simulink model "bObserver"  (R2020a)
settings: Solver=VariableStepAuto  StartTime=0.0  StopTime=1.5  FixedStep=0.0005  EnableMultiTasking=on
InitFcn:
  | kp=0.01;
  | ki=0.01;
  | 
  | k=2;
  | em=100000000;
  | GE=1/em;
  | GU=k*ki/GE;
  | GCE=k*kp/GU;
model workspace (MAT data in the model file):
  time = 0.8
values from neighbouring files (symbols this model uses):
  A1 = obj.boostConverter.A1    [BoostController.m]    (also in BoostConverter.m = [-obj.R/obj.L 0;0 -1/(obj.Ro*obj.C)]; BuckBoostConverter.m = [-obj.R/obj.L 0;0 -1/(obj.Ro*obj.C)]; obsmc.m = Asigma{1,1}; workspace_atual.mat = [-16.4  0; 0  -3.50877192982])
  A2 = obj.boostConverter.A2    [BoostController.m]    (also in BoostConverter.m = [-obj.R/obj.L -1/obj.L;1/obj.C -1/(obj.Ro*obj.C)]; BuckBoostConverter.m = [-obj.R/obj.L 1/obj.L;-1/obj.C -1/(obj.Ro*obj.C)]; obsmc.m = Asigma{1,2}; workspace_atual.mat = [-16.4  -200; 350.877192982  -3.50877192982])
  AlarmDeadTime = 0.50    (= 0.5)    [BoostFaultSimulation.m]    (also in workspace_atual.mat; workspace_certo.mat)
  B1 = obj.boostConverter.B1    [BoostController.m]    (also in BoostConverter.m = [1/obj.L;0]; BuckBoostConverter.m = [1/obj.L;0]; obsmc.m = Bsigma{1,1}; workspace_atual.mat = [200 0])
  B1f = [200 0]    [workspace_atual.mat]    (also in workspace_certo.mat)
  B2 = obj.boostConverter.B2    [BoostController.m]    (also in BoostConverter.m = obj.B1; obsmc.m = Bsigma{1,2}; workspace_atual.mat = [200 0]; workspace_certo.mat = [200 0])
  B2f = [200 0]    [workspace_atual.mat]    (also in workspace_certo.mat)
  boost_Amatrices = cat(3,obj.A1,obj.A2)    [BoostConverter.m]    (also in BuckBoostConverter.m; boostResults2Latex.m = boost.A_matrices(); workspace_atual.mat = [-16.4 0 0 -3.50877192982 -16.4 350.877192982 -200 -3.508771; workspace_certo.mat = [-16.4 0 0 -3.50877192982 -16.4 350.877192982 -200 -3.508771)
  boost_parameters = [obj.Ro,obj.R,obj.L,obj.C,obj.u]'    [BoostConverter.m]    (also in BuckBoostConverter.m; boostResults2Latex.m = boost.parameters(); workspace_atual.mat = [100 0.082 0.005 0.00285 190]; workspace_certo.mat = [100 0.082 0.005 0.00285 190])
  C = 1e-3    (= 0.001)    [boostResults2Latex.m]
  CiL = [0 1]    [workspace_atual.mat]    (also in workspace_certo.mat)
  Cmatrix = [1  0; 0  1]    [workspace_atual.mat]    (also in workspace_certo.mat)
  CVc = [1 0]    [workspace_atual.mat]    (also in workspace_certo.mat)
  D1 = [1  0; 0  1]    [workspace_atual.mat]    (also in workspace_certo.mat)
  F_11 = -16.4    [workspace_atual.mat]    (also in workspace_certo.mat)
  F_12 = -4812476.87956    [workspace_atual.mat]    (also in workspace_certo.mat)
  F_21 = -3.50877192982    [workspace_atual.mat]    (also in workspace_certo.mat)
  F_22 = -2.00703596657    [workspace_atual.mat]    (also in workspace_certo.mat)
  FaultClass = 0    [BoostFaultSimulation.m]    (also in workspace_atual.mat = 1; workspace_certo.mat = 1)
  H_1 = 13715.5123667    [workspace_atual.mat]    (also in workspace_certo.mat)
  iLFaultSwitch = 0    [BoostFaultSimulation.m]    (also in workspace_atual.mat; workspace_certo.mat)
  iLFaultTime = 1.70    (= 1.7)    [BoostFaultSimulation.m]    (also in workspace_atual.mat; workspace_certo.mat)
  iLGainFaultFactor = 15    [BoostFaultSimulation.m]    (also in workspace_atual.mat; workspace_certo.mat)
  iLNoiseFaultSwitch = 0    [BoostFaultSimulation.m]    (also in workspace_atual.mat; workspace_certo.mat)
  iLNoiseTime = 1.70    (= 1.7)    [BoostFaultSimulation.m]    (also in workspace_atual.mat; workspace_certo.mat)
  Jth = 2000    [workspace_atual.mat]    (also in workspace_certo.mat)
  L = 1e-3    (= 0.001)    [boostResults2Latex.m]    (also in obsmc.m = sdpvar(3,1,'full'))
  L_11 = -176809.798019    [workspace_atual.mat]    (also in workspace_certo.mat)
  L_12 = -66005538231.6    [workspace_atual.mat]    (also in workspace_certo.mat)
  L_21 = 0.0967961040176    [workspace_atual.mat]    (also in workspace_certo.mat)
  L_22 = 350.985265141    [workspace_atual.mat]    (also in workspace_certo.mat)
  LoadAddSignalSwitch = 1    [BoostFaultSimulation.m]    (also in workspace_atual.mat; workspace_certo.mat)
  LoadAddSwitch = 0    [BoostFaultSimulation.m]    (also in workspace_atual.mat; workspace_certo.mat)
  LoadAddTime = 0.90    (= 0.9)    [BoostFaultSimulation.m]    (also in workspace_atual.mat; workspace_certo.mat)
  LoadRemoveSignalSwitch = 1    [BoostFaultSimulation.m]    (also in workspace_atual.mat; workspace_certo.mat)
  LoadRemoveSwitch = 0    [BoostFaultSimulation.m]    (also in workspace_atual.mat; workspace_certo.mat)
  LoadRemoveTime = 0.90    (= 0.9)    [BoostFaultSimulation.m]    (also in workspace_atual.mat; workspace_certo.mat)
  LobsiL = [1737913.15707 66180.0912281]    [workspace_atual.mat]    (also in workspace_certo.mat)
  LobsVc = [61200 1]    [workspace_atual.mat]    (also in workspace_certo.mat)
  ObsEp = 70    [workspace_atual.mat]    (also in workspace_certo.mat)
  P = value(P)    [BoostController.m]    (also in boostResults2Latex.m = boost.calculateP(); obsmc.m = blkdiag(1/deltaAtilde(1,2),-1/deltaAtilde(2,1),1); workspace_atual.mat = [0.00235275094895  5.25738510027e-05; 5.25738510027e-05  0.0; workspace_certo.mat = [0.00235275094893  5.25738512446e-05; 5.25738512446e-05  0.0)
  Q_1 = [13715.5123667  1; 1  0]    [workspace_atual.mat]    (also in workspace_certo.mat)
  Q_2 = [1  0; 0.00750867981628  1]    [workspace_atual.mat]    (also in workspace_certo.mat)
  R = 0.1    [boostResults2Latex.m]    (also in workspace_atual.mat = 0.082; workspace_certo.mat = 0.082)
  ReconfigSwitch = 0    [BoostFaultSimulation.m]    (also in workspace_atual.mat; workspace_certo.mat)
  ReconfigTime = 1.707    [BoostFaultSimulation.m]    (also in workspace_atual.mat; workspace_certo.mat)
  rho = 5    [workspace_atual.mat]    (also in workspace_certo.mat)
  RMSfrequency = 47.61    [BoostFaultSimulation.m]    (also in workspace_atual.mat; workspace_certo.mat)
  Ro = 100    [BoostFaultSimulation.m]    (also in boostResults2Latex.m = 10; workspace_atual.mat; workspace_certo.mat)
  Smep = 80    [workspace_atual.mat]    (also in workspace_certo.mat)
  SourceAddSignalSwitch = 1    [BoostFaultSimulation.m]    (also in workspace_atual.mat; workspace_certo.mat)
  SourceAddSwitch = 0    [BoostFaultSimulation.m]    (also in workspace_atual.mat; workspace_certo.mat)
  SourceAddTime = 0.90    (= 0.9)    [BoostFaultSimulation.m]    (also in workspace_atual.mat; workspace_certo.mat)
  SourceAddVoltage = obj.SourceAddFactor*obj.u    [BoostFaultSimulation.m]    (also in workspace_atual.mat = 19; workspace_certo.mat = 19)
  SourceRemoveSignalSwitch = 1    [BoostFaultSimulation.m]    (also in workspace_atual.mat; workspace_certo.mat)
  SourceRemoveSwitch = 0    [BoostFaultSimulation.m]    (also in workspace_atual.mat; workspace_certo.mat)
  SourceRemoveTime = 0.90    (= 0.9)    [BoostFaultSimulation.m]    (also in workspace_atual.mat; workspace_certo.mat)
  SourceRemoveVoltage = obj.SourceRemoveFactor*obj.u    [BoostFaultSimulation.m]    (also in workspace_atual.mat = 19; workspace_certo.mat = 19)
  T_1 = [1 -13715.5123667]    [workspace_atual.mat]    (also in workspace_certo.mat)
  T_2 = [-0.00750867981628 1]    [workspace_atual.mat]    (also in workspace_certo.mat)
  ueq = 0.5    [workspace_atual.mat]    (also in workspace_certo.mat)
  uf = 190    [workspace_atual.mat]    (also in workspace_certo.mat)
  VcFaultSwitch = 0    [BoostFaultSimulation.m]    (also in workspace_atual.mat; workspace_certo.mat)
  VcFaultTime = 1.70    (= 1.7)    [BoostFaultSimulation.m]    (also in workspace_atual.mat; workspace_certo.mat)
  VcGainFaultFactor = 15    [BoostFaultSimulation.m]    (also in workspace_atual.mat; workspace_certo.mat)
  VcNoiseFaultSwitch = 0    [BoostFaultSimulation.m]    (also in workspace_atual.mat; workspace_certo.mat)
  VcNoiseTime = 1.70    (= 1.7)    [BoostFaultSimulation.m]    (also in workspace_atual.mat; workspace_certo.mat)
  ve = 380    [BoostFaultSimulation.m]    (also in boostResults2Latex.m = 100; workspace_atual.mat; workspace_certo.mat)
  x_e = [ie;ve]    [BoostConverter.m]    (also in BuckBoostConverter.m)
  xe = obj.boostConverter.equilibriumstate(ve)    [BoostController.m]    (also in workspace_atual.mat = [7.62509288104 380]; workspace_certo.mat = [7.62509288104 380])
undefined symbols (not defined in the file or in its folder): Atilde1, Atilde2, B1u, Ctilde1, Dtilde1, Dtilde2, F, F1, G, G1, MAXnet, MINnet
libraries: neural x36, powerlib x34, dspstat3 x11, PhdLibrary x10, simulink x7, dspmtrx3 x6, powerlib_meascontrol x4, dspmathops x4
(part 2 of 6)

== system bObserver/ROSLSO/Controlador1 ==
  note: Sinal de controle
  note: Superfície
  note: Ponto de equilíbrio
  ve : Inport
  x : Inport  Port=2
  "    " : Constant  Value=ueq
  "    2" : Constant  Value=Smep
  Constant6 : Constant  Value=boost_parameters
  Demux1 : Demux  Outputs=2
  Demux2 : Demux  Outputs=2
  Gain : Gain  Gain=0.2
  Gain1 : Gain  Gain=2
  Gain3 : Gain  Gain=2.3
  Integrator1 : Integrator
  PWM : powerlib_meascontrol/Pulse & Signal Generators/PWM Generator (DC-DC)  Fsw=7000  Ts=0
  Scope : Scope
  SlidingSurface : Subsystem
  Sum : Sum  Inputs=|++
  Sum4 : Sum  Inputs=++|
  Sum5 : Sum  Inputs=-+|
  Sum6 : Sum  Inputs=-+|
  Sum9 : Sum  Inputs=|++
  xe : MATLAB Function  TreatAsAtomicUnit=on
  sigma : Outport
  i_e : Outport  Port=2
  x_e : Outport  Port=3
  wires:
  Demux1/1 -> Sum6/2  "IL"
  PWM/1 -> sigma/1
  ve/1 -> xe/2(ve)
  Demux2/2 -> Sum5/1  "Vo1"
  "    "/1 -> Sum9/2
  Sum5/1 -> Gain3/1, Gain/1
  Sum9/1 -> PWM/1
  Demux1/2 -> Sum5/2  "Vo1"
  Demux2/1 -> Sum6/1
  xe/2(i_e) -> i_e/1
  x/1 -> Demux2/1
  Constant6/1 -> xe/1(boost_parameters)
  Gain1/1 -> Sum4/2
  xe/1(x_e) -> Demux1/1, x_e/1
  Gain/1 -> Sum/1
  Sum/1 -> Sum4/1
  SlidingSurface/1(d) -> Scope/1, Sum9/1
  "    2"/1 -> SlidingSurface/2(ep)
  Sum6/1 -> Gain1/1
  Gain3/1 -> Integrator1/1
  Sum4/1 -> SlidingSurface/1(S)

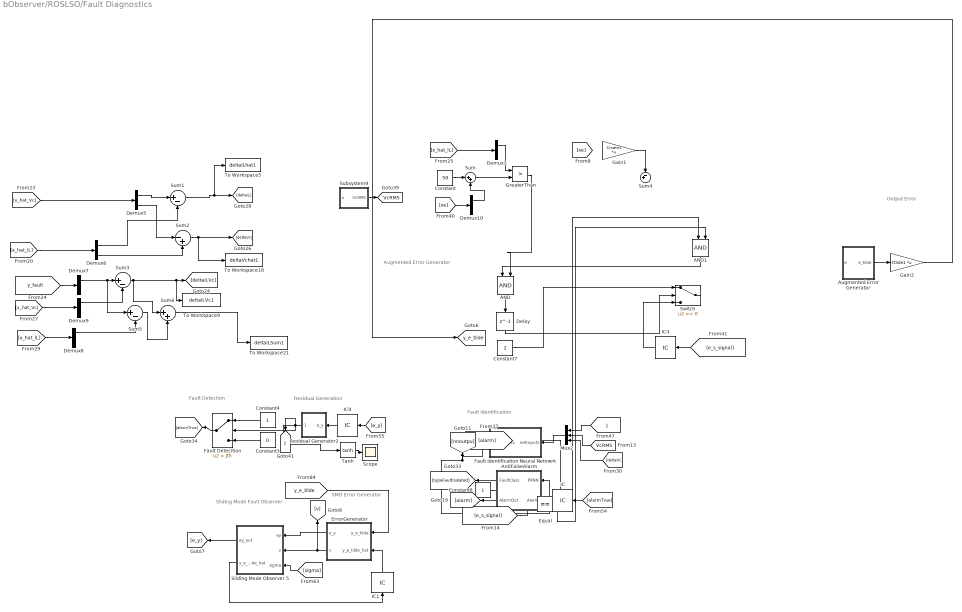
== system bObserver/ROSLSO/Fault Diagnostics ==
  note: Sliding Mode
      | Fault Observer
  note: SMO Error
      | Generator
  note: Residual Generation
  note: Fault identification
  note: Fault Detection
  note: Augmented Error Generator
  note: Output Error
  AND : Logic  IconShape=distinctive  AllPortsSameDT=off  OutDataTypeStr=boolean
  AND1 : Logic  IconShape=distinctive  AllPortsSameDT=off  OutDataTypeStr=boolean
  AntiFalseAlarm : Subsystem
  Augmented Error Generator : Subsystem
  Constant : Constant  Value=50
  Constant3 : Constant  Value=0
  Constant4 : Constant
  Constant7 : Constant  Value=2
  Constant8 : Constant
  Delay : Delay  DelayLength=1
  Demux{3,5..10} (7 alike) : Demux  Outputs=2
  Equal : RelationalOperator  Operator===  OutDataTypeStr=boolean  RndMeth=Simplest
  ErrorGenerator : Subsystem
  Fault Detecition : Switch  Criteria=u2 > Threshold  Threshold=Jth  ZeroCross=off
  Fault Identification Neural Netowrk : Subsystem
  Gain1 : Gain  Gain=Cmatrix  Multiplication=Matrix(K*u)
  Gain2 : Gain  Gain=Ctilde1  Multiplication=Matrix(K*u)
  GreaterThan : RelationalOperator  Operator=>  OutDataTypeStr=boolean  RndMeth=Simplest
  IC : InitialCondition  Value=0
  IC1 : InitialCondition  Value=[0;0]
  IC4 : InitialCondition
  IC9 : InitialCondition  Value=[0;0]
  Mux2 : Mux  Inputs=3
  Residual Generator2 : Subsystem
  Scope : Scope
  Sliding Mode Observer 5 : Subsystem
  Subsystem9 : Subsystem
  Sum : Sum  Inputs=|++
  Sum1 : Sum  Inputs=|+-
  Sum2 : Sum  Inputs=|-+
  Sum3 : Sum  Inputs=|+-
  Sum4 : Sum  Inputs=-+|
  Sum5 : Sum  Inputs=|+-
  Sum6 : Sum  Inputs=|++
  Switch : Switch
  Tanh : Trigonometry  Operator=tanh
  To Workspace18 : ToWorkspace  VariableName=deltaVchat1  SaveFormat=Timeseries  SampleTime=-1
  To Workspace21 : ToWorkspace  VariableName=deltaiLSum1  SaveFormat=Timeseries  SampleTime=-1
  To Workspace5 : ToWorkspace  VariableName=deltaiLhat1  SaveFormat=Timeseries  SampleTime=-1
  To Workspace9 : ToWorkspace  VariableName=deltaiLVc1  SaveFormat=Timeseries  SampleTime=-1
  tag scope: J=global, VcRMS=global, y_e_tilde=global
  wires:
  Residual Generator2/1(RMS) -> Fault Detecition/2, [J], Tanh/1
  AntiFalseAlarm/1(FaultClass) -> [typeFaultIsolated]
  [J] -> Mux2/1
  Sliding Mode Observer 5/1(ey_out) -> [e_y]
  Fault Identification Neural Netowrk/1(netOutputs) -> AntiFalseAlarm/1(PRNN), [nnoutpu]
  Tanh/1 -> Scope/1
  [alarmTrue] -> IC/1
  Constant4/1 -> Fault Detecition/1
  AntiFalseAlarm/2(AlarmOut) -> [alarm]
  ErrorGenerator/2(v) -> Sliding Mode Observer 5/2(v), [v]
  ErrorGenerator/1(e_y) -> Sliding Mode Observer 5/1(ey)
  [sigma] -> Sliding Mode Observer 5/3(sigma)
  [VcRMS] -> Mux2/2
  [deltaVc] -> Mux2/3
  Constant3/1 -> Fault Detecition/3
  [y_e_tilde] -> ErrorGenerator/1(y_e_tilde)
  Fault Detecition/1 -> [alarmTrue]
  Sliding Mode Observer 5/2(y_e_tilde_hat) -> IC1/1
  Mux2/1 -> Fault Identification Neural Netowrk/1(netInputs)
  IC/1 -> AntiFalseAlarm/2(Alarm)
  IC1/1 -> ErrorGenerator/2(y_e_tilde_hat)
  [e_y] -> IC9/1
  IC9/1 -> Residual Generator2/1(e_y)
  Augmented Error Generator/1(e_tilde) -> Gain2/1
  Gain2/1 -> [y_e_tilde]
  [x_hat_iL] -> Demux8/1
  Sum3/1 -> To Workspace9/1, [deltaiLVc], Sum6/1
  Demux8/1 -> Sum5/2
  [x_hat_Vc] -> Demux5/1
  [y_fault] -> Demux7/1
  Sum6/1 -> To Workspace21/1
  Demux9/1 -> Sum3/2
  Sum5/1 -> Sum6/2
  Demux7/1 -> Sum5/1, Sum3/1
  Sum1/1 -> To Workspace5/1, [deltaiL]
  Demux5/1 -> Sum1/1
  Sum2/1 -> To Workspace18/1, [deltaVc]
  [x_hat_Vc] -> Demux9/1
  Demux5/2 -> Sum2/1
  Demux6/1 -> Sum1/2
  Demux6/2 -> Sum2/2
  [x_hat_iL] -> Demux6/1
  GreaterThan/1 -> AND/2
  AND1/1 -> AND/1
  [e_s_signal] -> IC4/1
  [x_hat_iL] -> Demux3/1
  [alarm] -> AND1/1
  Demux10/1 -> Sum/2
  [e_s_signal] -> Equal/2
  Equal/1 -> AND1/2
  Constant/1 -> Sum/1
  Constant7/1 -> Switch/1
  Sum/1 -> GreaterThan/2
  IC4/1 -> Switch/3
  Demux3/1 -> GreaterThan/1
  Constant8/1 -> Equal/1
  [xe] -> Demux10/1
  AND/1 -> Delay/1
  Delay/1 -> Switch/2
  Subsystem9/1(VcRMS) -> [VcRMS]
  Gain1/1 -> Sum4/1
  ? -> Sum4/2

== system bObserver/ROSLSO/If Action Subsystem ==
  In1 : Inport
  Action Port : ActionPort  ActionPortLabel=case [ 0 ]:
  Out1 : Outport
  wires:
  In1/1 -> Out1/1

== system bObserver/ROSLSO/If Action Subsystem1 ==
  In1 : Inport
  Action Port : ActionPort  ActionPortLabel=default:
  Out1 : Outport
  wires:
  In1/1 -> Out1/1

== system bObserver/ROSLSO/If Action Subsystem2 ==
  y : Inport
  Action Port : ActionPort  ActionPortLabel=case [ 2 ]:
  x_hat : Outport
  wires:
  y/1 -> x_hat/1

== system bObserver/ROSLSO/If Action Subsystem4 ==
  y : Inport
  Action Port : ActionPort  ActionPortLabel=case [ 1 ]:
  x_hat : Outport
  wires:
  y/1 -> x_hat/1

== system bObserver/ROSLSO/Subsystem1 ==
  y : Inport
  Matrizes A1 : Constant  Value=CVc  VectorParams1D=off
  Matrizes A2 : Constant  Value=CiL  VectorParams1D=off
  Product : Product  Multiplication=Matrix(*)
  Product1 : Product  Multiplication=Matrix(*)
  y_f1 : Outport
  y_f2 : Outport  Port=2
  wires:
  y/1 -> Product1/2, Product/2
  Matrizes A2/1 -> Product/1
  Matrizes A1/1 -> Product1/1
  Product/1 -> y_f1/1
  Product1/1 -> y_f2/1

== system bObserver/ROSMO_L1/Augmented Error Generator ==
  y_fault : Inport
  xe : Inport  Port=2
  Gain1 : Gain  Gain=Cmatrix  Multiplication=Matrix(K*u)
  Gain2 : Gain  Gain=Ctilde1  Multiplication=Matrix(K*u)
  Mux : Mux  Inputs=2
  Sum4 : Sum  Inputs=-+|
  z1 : Subsystem
  e_tilde : Outport
  y_e_tilde : Outport  Port=2
  wires:
  z1/1(z) -> Mux/2
  Mux/1 -> Gain2/1, e_tilde/1
  Gain2/1 -> y_e_tilde/1
  xe/1 -> Gain1/1
  Gain1/1 -> Sum4/1
  y_fault/1 -> Sum4/2
  Sum4/1 -> Mux/1, z1/1(z_dot)

== system bObserver/ROSMO_L1/Boost Converter ==
  sigma : Inport
  u : Inport  Port=2
  Constant2 : Constant  Value=B1  VectorParams1D=off
  Constant4 : Constant  Value=A1  VectorParams1D=off
  Constant5 : Constant  Value=A2  VectorParams1D=off
  Gain : Gain  Gain=Cmatrix  Multiplication=Matrix(K*u)
  Integral : Subsystem
  Matrix Multiply : Product  Multiplication=Matrix(*)
  Matrix Multiply1 : Product  Multiplication=Matrix(*)
  Matrix Multiply2 : Product  Multiplication=Matrix(*)
  Sum : Sum  Inputs=|++
  Sum1 : Sum  Inputs=|++
  Switch1 : Switch  Criteria=u2 ~= 0
  x : Outport
  y : Outport  Port=2
  wires:
  [A1x] -> Sum/1
  [x] -> Matrix Multiply2/2, Matrix Multiply/2
  [Bu] -> Sum1/2
  [Bu] -> Sum/2
  Constant5/1 -> Matrix Multiply2/1
  Constant4/1 -> Matrix Multiply/1
  Matrix Multiply2/1 -> [A2x]
  [sys1] -> Switch1/1
  Matrix Multiply/1 -> [A1x]
  Sum/1 -> [sys1]
  Sum1/1 -> [sys2]
  [sys2] -> Switch1/3
  Switch1/1 -> Integral/1(x_dot)  "x"
  [A2x] -> Sum1/1
  sigma/1 -> Switch1/2
  Constant2/1 -> Matrix Multiply1/1
  Matrix Multiply1/1 -> [Bu]
  u/1 -> Matrix Multiply1/2
  Integral/1(x) -> Gain/1, x/1, [x]
  Gain/1 -> y/1

== system bObserver/ROSMO_L1/Controlador2 ==
  note: Sinal de controle
  note: Superfície
  xe : Inport
  x : Inport  Port=2
  "    " : Constant  Value=ueq
  "    2" : Constant  Value=Smep
  Demux1 : Demux  Outputs=2
  Demux2 : Demux  Outputs=2
  Gain : Gain  Gain=KVc
  Gain1 : Gain  Gain=KiL
  Gain3 : Gain  Gain=KiVc
  Integrator1 : Integrator
  PWM : powerlib_meascontrol/Pulse & Signal Generators/PWM Generator (DC-DC)  Fsw=Freq  Ts=0
  SlidingSurface : Subsystem
  Sum : Sum  Inputs=|++
  Sum4 : Sum  Inputs=++|
  Sum5 : Sum  Inputs=-+|
  Sum6 : Sum  Inputs=-+|
  Sum9 : Sum  Inputs=|++
  sigma : Outport
  d : Outport  Port=2
  wires:
  Demux1/1 -> Sum6/2  "IL"
  PWM/1 -> sigma/1
  Demux2/2 -> Sum5/1  "Vo1"
  "    "/1 -> Sum9/2
  Sum5/1 -> Gain3/1, Gain/1
  Sum9/1 -> PWM/1
  Demux1/2 -> Sum5/2  "Vo1"
  Demux2/1 -> Sum6/1
  x/1 -> Demux2/1
  Gain1/1 -> Sum4/2
  Gain/1 -> Sum/1
  Sum/1 -> Sum4/1
  SlidingSurface/1(d) -> d/1, Sum9/1
  "    2"/1 -> SlidingSurface/2(ep)
  Sum6/1 -> Gain1/1
  Gain3/1 -> Integrator1/1
  Sum4/1 -> SlidingSurface/1(S)
  Integrator1/1 -> Sum/2
  xe/1 -> Demux1/1

== system bObserver/ROSMO_L1/Residual Generator2 ==
  e_y : Inport
  Matrix Square1 : dspmtrx3/Matrix Square  OutMin=[]  OutMax=[]
      settings: SourceProductBaseCode=DS
  Moving RMS : dspstat3/Moving RMS  Method=Sliding window  ForgettingFactorPort=off  SpecifyWindowLength=on  WindowLength=RMSfrequency/10  ForgettingFactor=0.9  SimulateUsing=Code generation
      settings: SourceProductBaseCode=DS
  Sqrt2 : Sqrt  SaturateOnIntegerOverflow=on
  RMS : Outport
  wires:
  Matrix Square1/1 -> Sqrt2/1
  Sqrt2/1 -> Moving RMS/1
  Moving RMS/1 -> RMS/1
  e_y/1 -> Matrix Square1/1

== system bObserver/ROSMO_L1/SMO ==
  y_e_tilde : Inport
  sigma : Inport  Port=2
  ErrorGenerator : Subsystem
  IC2 : InitialCondition  Value=[0;0]
  Sliding Mode Observer 5 : Subsystem
  e_y : Outport
  v : Outport  Port=2
  wires:
  Sliding Mode Observer 5/1(ey_out) -> e_y/1
  Sliding Mode Observer 5/2(y_e_tilde_hat) -> IC2/1
  ErrorGenerator/2(v) -> v/1, Sliding Mode Observer 5/2(v)
  ErrorGenerator/1(e_y) -> Sliding Mode Observer 5/1(ey)
  IC2/1 -> ErrorGenerator/2(y_e_tilde_hat)
  y_e_tilde/1 -> ErrorGenerator/1(y_e_tilde)
  sigma/1 -> Sliding Mode Observer 5/3(sigma)

== system bObserver/ROSMO_L1/Subsystem ==
  y : Inport
  faultType : Inport  Port=2
  Constant4 : Constant  Value=[iLfgain;0]  VectorParams1D=off
  Constant7 : Constant  Value=[0;Vcfgain]  VectorParams1D=off
  Constant8 : Constant  Value=[0;0]  VectorParams1D=off
  Sum : Sum  Inputs=|++
  iLFault Switch : MultiPortSwitch  DataPortOrder=Zero-based contiguous  DataPortForDefault=Additional data port  zeroidx=on
  y_fault : Outport
  wires:
  y/1 -> Sum/2
  Constant8/1 -> iLFault Switch/5, iLFault Switch/2
  iLFault Switch/1 -> Sum/1
  Constant7/1 -> iLFault Switch/4
  Constant4/1 -> iLFault Switch/3
  faultType/1 -> iLFault Switch/1
  Sum/1 -> y_fault/1

== system bObserver/ROSMO_ROSLSO/Augmented Error Generator ==
  y_fault : Inport
  xe : Inport  Port=2
  Gain1 : Gain  Gain=Cmatrix  Multiplication=Matrix(K*u)
  Gain2 : Gain  Gain=Ctilde1  Multiplication=Matrix(K*u)
  Mux : Mux  Inputs=2
  Sum4 : Sum  Inputs=-+|
  z1 : Subsystem
  e_tilde : Outport
  y_e_tilde : Outport  Port=2
  wires:
  z1/1(z) -> Mux/2
  Mux/1 -> Gain2/1, e_tilde/1
  Gain2/1 -> y_e_tilde/1
  xe/1 -> Gain1/1
  Gain1/1 -> Sum4/1
  y_fault/1 -> Sum4/2
  Sum4/1 -> Mux/1, z1/1(z_dot)

== system bObserver/ROSMO_ROSLSO/Bank of ROSLSO ==
  y_f0 : Inport
  y_f1 : Inport  Port=2
  y_f2 : Inport  Port=3
  sigma : Inport  Port=4
  Constant : Constant  Value=uf  VectorParams1D=off
  ROSLSO 2 Subsystems : Subsystem  mask(ROSLSO){B1=B1f, B2=B2f, T=T_1, F1=F_11, F2=F_12, L1=L_11, L2=L_12, Q=Q_1, z0=0}
      mask prompts: B1 "Input matrix system 1:"; B2 "Input matrix system 2:"; T "Input gain matrix:"; F1 "Observer matrix system 1:"; F2 "Observer matrix system 2:"; L1 "Output gain matrix system 1:"; L2 "Output gain matrix system 2:"; Q "Weight matrix"; z0 "Initial conditions:"
      mask help:
      | Reduced Order Switched Linear Systems Observer
      | Estimates only the unmensured variables and concatenate with output
  ROSLSO 2 Subsystems1 : Subsystem  mask(ROSLSO){B1=B1f, B2=B2f, T=T_2, F1=F_21, F2=F_22, L1=L_21, L2=L_22, Q=Q_2, z0=0}
      mask prompts: B1 "Input matrix system 1:"; B2 "Input matrix system 2:"; T "Input gain matrix:"; F1 "Observer matrix system 1:"; F2 "Observer matrix system 2:"; L1 "Output gain matrix system 1:"; L2 "Output gain matrix system 2:"; Q "Weight matrix"; z0 "Initial conditions:"
      mask help:
      | Reduced Order Switched Linear Systems Observer
      | Estimates only the unmensured variables and concatenate with output
  Terminator : Terminator
  Terminator1 : Terminator
  x_hat_iL : Outport
  x_hat_Vc : Outport  Port=2
  x_hat_0 : Outport  Port=3
  wires:
  sigma/1 -> ROSLSO 2 Subsystems/3(sigma), ROSLSO 2 Subsystems1/3(sigma)
  y_f1/1 -> ROSLSO 2 Subsystems/2(y)
  y_f2/1 -> ROSLSO 2 Subsystems1/2(y)
  Constant/1 -> ROSLSO 2 Subsystems/1(u), ROSLSO 2 Subsystems1/1(u)
  ROSLSO 2 Subsystems1/2(xhat) -> x_hat_Vc/1
  ROSLSO 2 Subsystems/2(xhat) -> x_hat_iL/1
  ROSLSO 2 Subsystems/1(z) -> Terminator/1
  ROSLSO 2 Subsystems1/1(z) -> Terminator1/1
  y_f0/1 -> x_hat_0/1

== system bObserver/ROSMO_ROSLSO/Boost Converter ==
  sigma : Inport
  u : Inport  Port=2
  Constant2 : Constant  Value=B1  VectorParams1D=off
  Constant4 : Constant  Value=A1  VectorParams1D=off
  Constant5 : Constant  Value=A2  VectorParams1D=off
  Gain : Gain  Gain=Cmatrix  Multiplication=Matrix(K*u)
  Integral : Subsystem
  Matrix Multiply : Product  Multiplication=Matrix(*)
  Matrix Multiply1 : Product  Multiplication=Matrix(*)
  Matrix Multiply2 : Product  Multiplication=Matrix(*)
  Sum : Sum  Inputs=|++
  Sum1 : Sum  Inputs=|++
  Switch1 : Switch  Criteria=u2 ~= 0
  x : Outport
  y : Outport  Port=2
  wires:
  [A1x] -> Sum/1
  [x] -> Matrix Multiply2/2, Matrix Multiply/2
  [Bu] -> Sum1/2
  [Bu] -> Sum/2
  Constant5/1 -> Matrix Multiply2/1
  Constant4/1 -> Matrix Multiply/1
  Matrix Multiply2/1 -> [A2x]
  [sys1] -> Switch1/1
  Matrix Multiply/1 -> [A1x]
  Sum/1 -> [sys1]
  Sum1/1 -> [sys2]
  [sys2] -> Switch1/3
  Switch1/1 -> Integral/1(x_dot)  "x"
  [A2x] -> Sum1/1
  sigma/1 -> Switch1/2
  Constant2/1 -> Matrix Multiply1/1
  Matrix Multiply1/1 -> [Bu]
  u/1 -> Matrix Multiply1/2
  Integral/1(x) -> Gain/1, x/1, [x]
  Gain/1 -> y/1

== system bObserver/ROSMO_ROSLSO/Boost Converter Circuit ==
  sigma : Inport
  Boost Converter Circuit : Subsystem  mask(Boost Converter circuit){R=R, c=C, l=L}
      mask prompts: R "Resistance"; c "Capacitance"; l "Indutance"
      mask help: Boost Converter circuit with nonideal switching (IGBT)
  Constant : Constant  Value=Cmatrix
  DC Source : Subsystem
  Matrix Multiply : Product  Multiplication=Matrix(*)
  Mux1 : Mux  Inputs=2
  Output Resistance : Subsystem
  Terminator : Terminator
  Terminator1 : Terminator
  Voltage Measurement1 : powerlib/Measurements/Voltage Measurement  PhasorSimulation=off  OutputType=Complex  PSBequivalent=0
  x : Outport
  y : Outport  Port=2
  wires:
  sigma/1 -> Boost Converter Circuit/1(sigma)
  Boost Converter Circuit/1(iL) -> Mux1/1
  Boost Converter Circuit/2(Vc) -> Mux1/2
  Mux1/1 -> Matrix Multiply/2, x/1
  Boost Converter Circuit/3(iro) -> Terminator/1
  Voltage Measurement1/1 -> Terminator1/1
  Constant/1 -> Matrix Multiply/1
  Matrix Multiply/1 -> y/1
  connections:
  DC Source/RConn1 -- Boost Converter Circuit/LConn1 -- Voltage Measurement1/LConn1
  DC Source/RConn2 -- Boost Converter Circuit/LConn2 -- Voltage Measurement1/LConn2
  Output Resistance/RConn1 -- Boost Converter Circuit/LConn3
  Output Resistance/RConn2 -- Boost Converter Circuit/LConn4

== system bObserver/ROSMO_ROSLSO/Controlador2 ==
  note: Sinal de controle
  note: Superfície
  xe : Inport
  x : Inport  Port=2
  "    " : Constant  Value=ueq
  Demux1 : Demux  Outputs=2
  Demux2 : Demux  Outputs=2
  Gain : Gain  Gain=KVc
  Gain1 : Gain  Gain=KiL
  Gain3 : Gain  Gain=KiVc
  Integrator1 : Integrator
  Limit Layer : PhdLibrary/Integral Sliding  Mode Controller/SlidingSurface  Smep=Smep
      settings: SourceProductName=Phd Diego
  PWM : powerlib_meascontrol/Pulse & Signal Generators/PWM Generator (DC-DC)  Fsw=Freq  Ts=0
  Sum : Sum  Inputs=|++
  Sum4 : Sum  Inputs=++|
  Sum5 : Sum  Inputs=-+|
  Sum6 : Sum  Inputs=-+|
  Sum9 : Sum  Inputs=|++
  sigma : Outport
  d : Outport  Port=2
  wires:
  Demux1/1 -> Sum6/2  "IL"
  PWM/1 -> sigma/1
  Demux2/2 -> Sum5/1  "Vo1"
  "    "/1 -> Sum9/2
  Sum5/1 -> Gain3/1, Gain/1
  Sum9/1 -> PWM/1
  Demux1/2 -> Sum5/2  "Vo1"
  Demux2/1 -> Sum6/1
  x/1 -> Demux2/1
  Gain1/1 -> Sum4/2
  Gain/1 -> Sum/1
  Sum/1 -> Sum4/1
  Limit Layer/1 -> d/1, Sum9/1
  Sum6/1 -> Gain1/1
  Gain3/1 -> Integrator1/1
  Integrator1/1 -> Sum/2
  xe/1 -> Demux1/1
  Sum4/1 -> Limit Layer/1

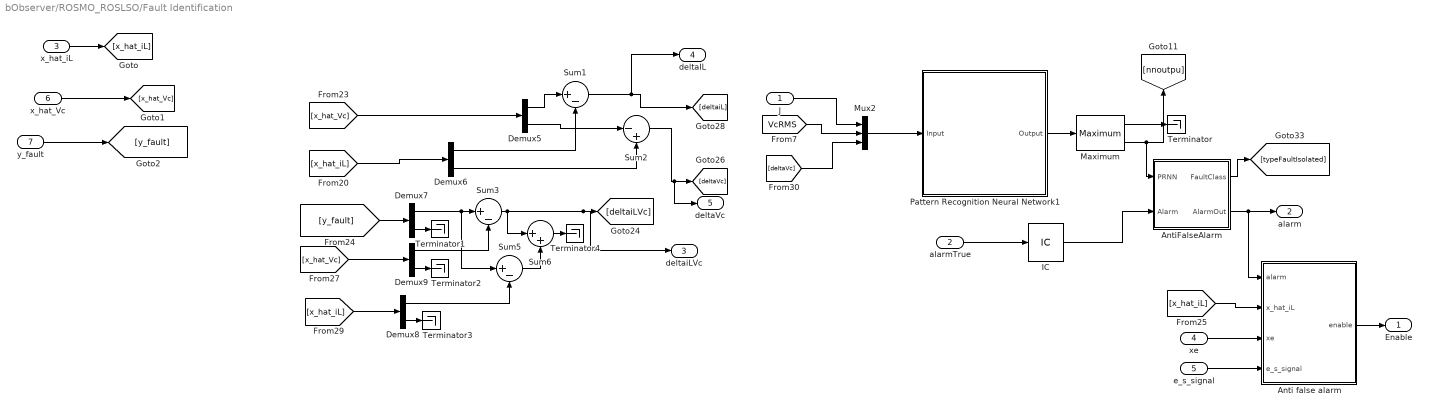
== system bObserver/ROSMO_ROSLSO/Fault Identification ==
  J : Inport
  alarmTrue : Inport  Port=2
  x_hat_iL : Inport  Port=3
  xe : Inport  Port=4
  e_s_signal : Inport  Port=5
  x_hat_Vc : Inport  Port=6
  y_fault : Inport  Port=7
  Anti false alarm : Subsystem
  AntiFalseAlarm : Subsystem
  Demux{5..9} (5 alike) : Demux  Outputs=2
  IC : InitialCondition  Value=0
  Maximum : dspstat3/Maximum  operation=maximum  fcn=Value and Index  indexBase=One  operateOver=Each column  Dimension=1  InputProcessing=Columns as channels (frame based)  reset=None  roiEnable=off  roiType=Rectangles  roiPortion=Entire ROI  roiOutput=Individual statistics for each ROI  roiFlag=off  roundingMode=Floor  overflowMode=off  accumDataTypeStr=Inherit: Same as product output  accumLastDataTypeStr=Inherit: Same as product output
  Mux2 : Mux  Inputs=3
  Pattern Recognition Neural Network1 : Subsystem
      mask help: Pattern Recognition Neural Network
      mask Display: e = 0.06;c1 = [120 150 230]/255;c2 = ([120 150 230]+0)/383;c3 = ([120 150 230]+128)/383;patch([0 1 1 0],[0 0 1 1],c1);patch([0 1 1 1-e 1-e 0+e],[0 0 1 1-e 0+e 0+e],c2);patch([0 0 1 1-e 0+e 0+e],[0 1 1 1-e 1-e 0+e],c3);plot([0 1 1 0 0],[0 0 1 1 0]);fprintf('NNET');port_label('input',1,' Input');port_label('output',1,'Output ');
  Sum1 : Sum  Inputs=|+-
  Sum2 : Sum  Inputs=|-+
  Sum3 : Sum  Inputs=|+-
  Sum5 : Sum  Inputs=|+-
  Sum6 : Sum  Inputs=|++
  Terminator{,1..4} (5 alike) : Terminator
  Enable : Outport
  alarm : Outport  Port=2
  deltaiLVc : Outport  Port=3
  deltaIL : Outport  Port=4
  deltaVc : Outport  Port=5
  wires:
  Demux6/2 -> Sum2/2
  Sum2/1 -> deltaVc/1, [deltaVc]
  Demux7/2 -> Terminator1/1
  Sum5/1 -> Sum6/2
  [y_fault] -> Demux7/1
  Sum3/1 -> deltaiLVc/1, [deltaiLVc], Sum6/1
  Demux5/2 -> Sum2/1
  [x_hat_Vc] -> Demux9/1
  Demux5/1 -> Sum1/1
  Demux9/1 -> Sum3/2
  [deltaVc] -> Mux2/3
  [x_hat_Vc] -> Demux5/1
  Demux6/1 -> Sum1/2
  Demux8/1 -> Sum5/2
  Demux7/1 -> Sum5/1, Sum3/1
  [VcRMS] -> Mux2/2
  [x_hat_iL] -> Demux6/1
  Sum1/1 -> deltaIL/1, [deltaiL]
  [x_hat_iL] -> Demux8/1
  Demux9/2 -> Terminator2/1
  Demux8/2 -> Terminator3/1
  J/1 -> Mux2/1
  Maximum/1 -> Terminator/1
  Pattern Recognition Neural Network1/1(Output) -> Maximum/1
  Mux2/1 -> Pattern Recognition Neural Network1/1(Input)
  Maximum/2 -> AntiFalseAlarm/1(PRNN), [nnoutpu]
  alarmTrue/1 -> IC/1
  IC/1 -> AntiFalseAlarm/2(Alarm)
  AntiFalseAlarm/1(FaultClass) -> [typeFaultIsolated]
  AntiFalseAlarm/2(AlarmOut) -> alarm/1, Anti false alarm/1(alarm)
  xe/1 -> Anti false alarm/3(xe)
  e_s_signal/1 -> Anti false alarm/4(e_s_signal)
  Anti false alarm/1(enable) -> Enable/1
  x_hat_iL/1 -> [x_hat_iL]
  [x_hat_iL] -> Anti false alarm/2(x_hat_iL)
  x_hat_Vc/1 -> [x_hat_Vc]
  y_fault/1 -> [y_fault]
  Sum6/1 -> Terminator4/1

== system bObserver/ROSMO_ROSLSO/Flawlesse Output Separator 2x1 ==
  y : Inport
  Matrizes A1 : Constant  Value=Cf2  VectorParams1D=off
  Matrizes A2 : Constant  Value=Cf1  VectorParams1D=off
  Product : Product  Multiplication=Matrix(*)
  Product1 : Product  Multiplication=Matrix(*)
  y_f1 : Outport
  y_f2 : Outport  Port=2
  wires:
  y/1 -> Product1/2, Product/2
  Matrizes A2/1 -> Product/1
  Matrizes A1/1 -> Product1/1
  Product/1 -> y_f1/1
  Product1/1 -> y_f2/1

== system bObserver/ROSMO_ROSLSO/Noise Fault Generator ==
  y : Inport
  faultType1 : Inport  Port=2
  Band-Limited White Noise1 : simulink/Sources/Band-Limited White Noise  Cov=[0.1]  Ts=0.1  seed=[23341]  VectorParams1D=off
  Constant2 : Constant  Value=[0 0;0 0]  VectorParams1D=off
  Constant5 : Constant  Value=[1 0;0 0]  VectorParams1D=off
  Constant6 : Constant  Value=[0 0;0 1]  VectorParams1D=off
  Matrix Multiply : Product  Multiplication=Matrix(*)
  Noise Fault Switch : MultiPortSwitch  DataPortOrder=Zero-based contiguous  DataPortForDefault=Additional data port  zeroidx=on
  Sum1 : Sum  Inputs=|++
  yfault : Outport
  wires:
  faultType1/1 -> Noise Fault Switch/1
  Constant5/1 -> Noise Fault Switch/3
  Constant6/1 -> Noise Fault Switch/4
  Band-Limited White Noise1/1 -> Matrix Multiply/2
  Noise Fault Switch/1 -> Matrix Multiply/1
  Constant2/1 -> Noise Fault Switch/5, Noise Fault Switch/2
  Sum1/1 -> yfault/1
  y/1 -> Sum1/2
  Matrix Multiply/1 -> Sum1/1

== system bObserver/ROSMO_ROSLSO/Residual Generator2 ==
  e_y : Inport
  Matrix Square1 : dspmtrx3/Matrix Square  OutMin=[]  OutMax=[]
      settings: SourceProductBaseCode=DS
  Moving RMS : dspstat3/Moving RMS  Method=Sliding window  ForgettingFactorPort=off  SpecifyWindowLength=on  WindowLength=RMSfrequency/10  ForgettingFactor=0.9  SimulateUsing=Code generation
      settings: SourceProductBaseCode=DS
  Sqrt2 : Sqrt  SaturateOnIntegerOverflow=on
  RMS : Outport
  wires:
  Matrix Square1/1 -> Sqrt2/1
  Sqrt2/1 -> Moving RMS/1
  Moving RMS/1 -> RMS/1
  e_y/1 -> Matrix Square1/1

== system bObserver/ROSMO_ROSLSO/SMO ==
  y_e_tilde : Inport
  sigma : Inport  Port=2
  ErrorGenerator : Subsystem
  IC2 : InitialCondition  Value=[0;0]
  Sliding Mode Observer 5 : Subsystem
  e_y : Outport
  v : Outport  Port=2
  wires:
  Sliding Mode Observer 5/1(ey_out) -> e_y/1
  Sliding Mode Observer 5/2(y_e_tilde_hat) -> IC2/1
  ErrorGenerator/2(v) -> v/1, Sliding Mode Observer 5/2(v)
  ErrorGenerator/1(e_y) -> Sliding Mode Observer 5/1(ey)
  IC2/1 -> ErrorGenerator/2(y_e_tilde_hat)
  y_e_tilde/1 -> ErrorGenerator/1(y_e_tilde)
  sigma/1 -> Sliding Mode Observer 5/3(sigma)

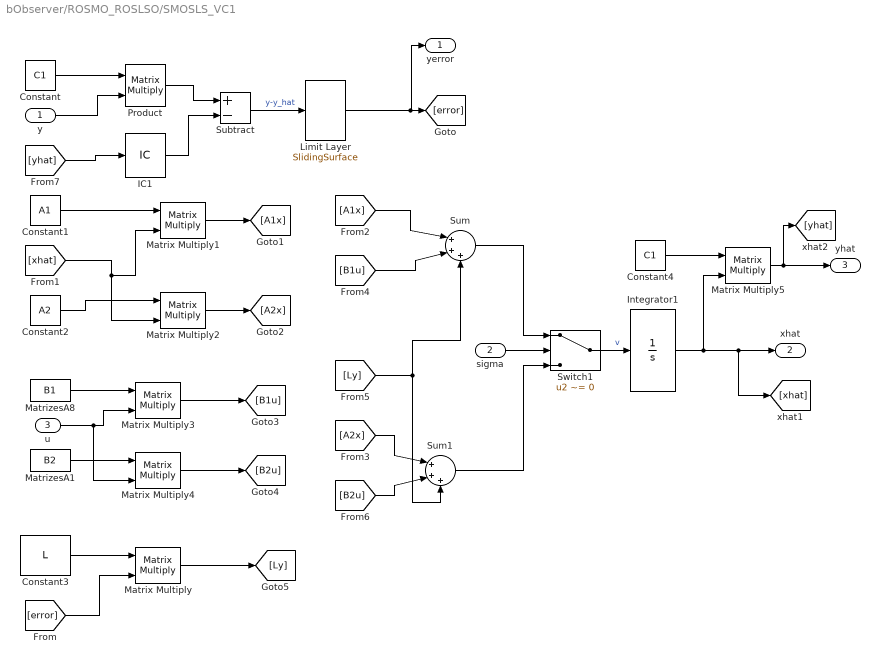
== system bObserver/ROSMO_ROSLSO/SMOSLS_VC1 ==
  y : Inport
  sigma : Inport  Port=2
  u : Inport  Port=3
  Constant : Constant  Value=C1  VectorParams1D=off
  Constant1 : Constant  Value=A1  VectorParams1D=off
  Constant2 : Constant  Value=A2  VectorParams1D=off
  Constant3 : Constant  Value=L  VectorParams1D=off
  Constant4 : Constant  Value=C1  VectorParams1D=off
  IC1 : InitialCondition  Value=yhat0
  Integrator1 : Integrator  InitialCondition=x0
  Limit Layer : PhdLibrary/Integral Sliding  Mode Controller/SlidingSurface  Smep=ObsEp
      settings: SourceProductName=Phd Diego
  Matrix Multiply{,1..5} (6 alike) : Product  Multiplication=Matrix(*)
  MatrizesA1 : Constant  Value=B2  VectorParams1D=off
  MatrizesA8 : Constant  Value=B1  VectorParams1D=off
  Product : Product  Multiplication=Matrix(*)
  Subtract : Sum  Inputs=+-
  Sum : Sum  Inputs=|+++
  Sum1 : Sum  Inputs=|+++
  Switch1 : Switch  Criteria=u2 ~= 0
  yerror : Outport
  xhat : Outport  Port=2
  yhat : Outport  Port=3
  wires:
  Subtract/1 -> Limit Layer/1  "y-y_hat"
  Product/1 -> Subtract/1
  Limit Layer/1 -> yerror/1, [error]
  [yhat] -> IC1/1
  y/1 -> Product/2
  Constant/1 -> Product/1
  Constant3/1 -> Matrix Multiply/1
  MatrizesA8/1 -> Matrix Multiply3/1
  Sum/1 -> Switch1/1
  [error] -> Matrix Multiply/2
  Constant1/1 -> Matrix Multiply1/1
  [B1u] -> Sum/2
  Matrix Multiply4/1 -> [B2u]
  [Ly] -> Sum/3, Sum1/3
  [A2x] -> Sum1/1
  [A1x] -> Sum/1
  [B2u] -> Sum1/2
  Matrix Multiply3/1 -> [B1u]
  u/1 -> Matrix Multiply4/2, Matrix Multiply3/2
  MatrizesA1/1 -> Matrix Multiply4/1
  sigma/1 -> Switch1/2
  Matrix Multiply1/1 -> [A1x]
  Sum1/1 -> Switch1/3
  Constant4/1 -> Matrix Multiply5/1
  Constant2/1 -> Matrix Multiply2/1
  Integrator1/1 -> xhat/1, [xhat], Matrix Multiply5/2
  Matrix Multiply5/1 -> [yhat], yhat/1
  Matrix Multiply2/1 -> [A2x]
  Switch1/1 -> Integrator1/1  "v"
  Matrix Multiply/1 -> [Ly]
  [xhat] -> Matrix Multiply2/2, Matrix Multiply1/2
  IC1/1 -> Subtract/2

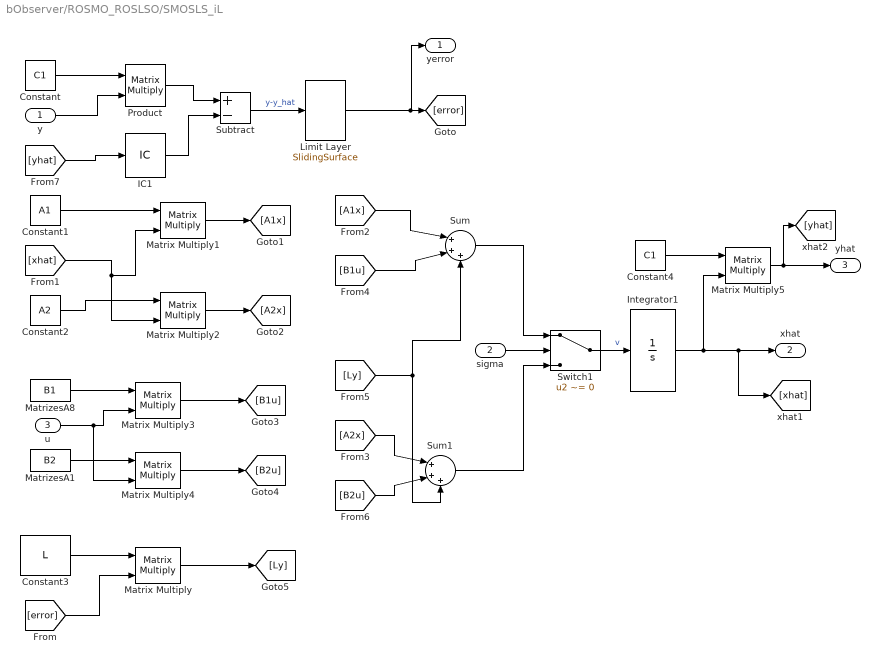
== system bObserver/ROSMO_ROSLSO/SMOSLS_iL ==
  y : Inport
  sigma : Inport  Port=2
  u : Inport  Port=3
  Constant : Constant  Value=C1  VectorParams1D=off
  Constant1 : Constant  Value=A1  VectorParams1D=off
  Constant2 : Constant  Value=A2  VectorParams1D=off
  Constant3 : Constant  Value=L  VectorParams1D=off
  Constant4 : Constant  Value=C1  VectorParams1D=off
  IC1 : InitialCondition  Value=yhat0
  Integrator1 : Integrator  InitialCondition=x0
  Limit Layer : PhdLibrary/Integral Sliding  Mode Controller/SlidingSurface  Smep=ObsEp
      settings: SourceProductName=Phd Diego
  Matrix Multiply{,1..5} (6 alike) : Product  Multiplication=Matrix(*)
  MatrizesA1 : Constant  Value=B2  VectorParams1D=off
  MatrizesA8 : Constant  Value=B1  VectorParams1D=off
  Product : Product  Multiplication=Matrix(*)
  Subtract : Sum  Inputs=+-
  Sum : Sum  Inputs=|+++
  Sum1 : Sum  Inputs=|+++
  Switch1 : Switch  Criteria=u2 ~= 0
  yerror : Outport
  xhat : Outport  Port=2
  yhat : Outport  Port=3
  wires:
  Subtract/1 -> Limit Layer/1  "y-y_hat"
  Product/1 -> Subtract/1
  Limit Layer/1 -> yerror/1, [error]
  [yhat] -> IC1/1
  y/1 -> Product/2
  Constant/1 -> Product/1
  Constant3/1 -> Matrix Multiply/1
  MatrizesA8/1 -> Matrix Multiply3/1
  Sum/1 -> Switch1/1
  [error] -> Matrix Multiply/2
  Constant1/1 -> Matrix Multiply1/1
  [B1u] -> Sum/2
  Matrix Multiply4/1 -> [B2u]
  [Ly] -> Sum/3, Sum1/3
  [A2x] -> Sum1/1
  [A1x] -> Sum/1
  [B2u] -> Sum1/2
  Matrix Multiply3/1 -> [B1u]
  u/1 -> Matrix Multiply4/2, Matrix Multiply3/2
  MatrizesA1/1 -> Matrix Multiply4/1
  sigma/1 -> Switch1/2
  Matrix Multiply1/1 -> [A1x]
  Sum1/1 -> Switch1/3
  Constant4/1 -> Matrix Multiply5/1
  Constant2/1 -> Matrix Multiply2/1
  Integrator1/1 -> xhat/1, [xhat], Matrix Multiply5/2
  Matrix Multiply5/1 -> [yhat], yhat/1
  Matrix Multiply2/1 -> [A2x]
  Switch1/1 -> Integrator1/1  "v"
  Matrix Multiply/1 -> [Ly]
  [xhat] -> Matrix Multiply2/2, Matrix Multiply1/2
  IC1/1 -> Subtract/2

== system bObserver/ROSMO_ROSLSO/Sensor Gain Fault Generator ==
  y : Inport
  faultType : Inport  Port=2
  Constant4 : Constant  Value=[1 0;0 1]  VectorParams1D=off
  Constant7 : Constant  Value=[s1gain 0;0 1]  VectorParams1D=off
  Constant8 : Constant  Value=[1 0;0 s2gain]  VectorParams1D=off
  Matrix Multiply : Product  Multiplication=Matrix(*)
  iLFault Switch : MultiPortSwitch  DataPortOrder=Zero-based contiguous  DataPortForDefault=Additional data port  zeroidx=on
  yfault : Outport
  wires:
  Matrix Multiply/1 -> yfault/1
  faultType/1 -> iLFault Switch/1
  Constant8/1 -> iLFault Switch/4
  iLFault Switch/1 -> Matrix Multiply/1
  Constant7/1 -> iLFault Switch/3
  Constant4/1 -> iLFault Switch/5, iLFault Switch/2
  y/1 -> Matrix Multiply/2

== system bObserver/Slding Mode/Anti false alarm ==
  x_hat_iL : Inport
  xe : Inport  Port=2
  alarm : Inport  Port=3
  e_s_signal : Inport  Port=4
  AND : Logic  IconShape=distinctive  AllPortsSameDT=off  OutDataTypeStr=boolean
  AND1 : Logic  IconShape=distinctive  AllPortsSameDT=off  OutDataTypeStr=boolean
  Constant : Constant  Value=50
  Constant7 : Constant  Value=2
  Constant8 : Constant
  Delay : Delay  DelayLength=1
  Demux10 : Demux  Outputs=2
  Demux3 : Demux  Outputs=2
  Equal : RelationalOperator  Operator===  OutDataTypeStr=boolean  RndMeth=Simplest
  GreaterThan : RelationalOperator  Operator=>  OutDataTypeStr=boolean  RndMeth=Simplest
  IC4 : InitialCondition
  Sum : Sum  Inputs=|++
  Switch : Switch
  Terminator : Terminator
  Terminator1 : Terminator
  enable : Outport
  wires:
  IC4/1 -> Switch/3
  [e_s_signal] -> IC4/1
  AND/1 -> Delay/1
  Constant/1 -> Sum/1
  AND1/1 -> AND/1
  Sum/1 -> GreaterThan/2
  GreaterThan/1 -> AND/2
  Delay/1 -> Switch/2
  Demux3/1 -> GreaterThan/1
  Constant8/1 -> Equal/1
  Equal/1 -> AND1/2
  Demux10/1 -> Sum/2
  Constant7/1 -> Switch/1
  Demux10/2 -> Terminator1/1
  x_hat_iL/1 -> Demux3/1
  Demux3/2 -> Terminator/1
  xe/1 -> Demux10/1
  alarm/1 -> AND1/1
  e_s_signal/1 -> [e_s_signal], Equal/2
  Switch/1 -> enable/1

== system bObserver/Slding Mode/AntiFalseAlarm ==
  PRNN : Inport
  Alarm : Inport  Port=2
  Constant7 : Constant
  FaultDetecition1 : Switch  Criteria=u2 > Threshold
  Product1 : Product
  Step1 : Step  Time=AlarmDeadTime  SampleTime=0
  FaultClass : Outport
  AlarmOut : Outport  Port=2
  wires:
  PRNN/1 -> FaultDetecition1/1
  Constant7/1 -> FaultDetecition1/3
  Step1/1 -> Product1/1
  Alarm/1 -> Product1/2
  FaultDetecition1/1 -> FaultClass/1
  Product1/1 -> AlarmOut/1, FaultDetecition1/2

== system bObserver/Slding Mode/Augmented Error Generator ==
  e : Inport
  Mux : Mux  Inputs=2
  z1 : Subsystem
  e_tilde : Outport
  wires:
  z1/1(z) -> Mux/2
  Mux/1 -> e_tilde/1
  e/1 -> Mux/1, z1/1(z_dot)

== system bObserver/Slding Mode/Boost Converter ==
  note: Escolha do tipo de entrada
  note: Circuito do conversor
  sigma : Inport
  ConversorBoost : Subsystem
  Mux1 : Mux  Inputs=2
  Terminator : Terminator
  Terminator1 : Terminator
  TipoEntrada : Subsystem
  x : Outport
  wires:
  TipoEntrada/4("Rvariavel ") -> [Rinput]
  sigma/1 -> ConversorBoost/1(sigma)
  [Vinput1] -> ?
  [Vinput2] -> ?
  [Rinput] -> ?
  TipoEntrada/5("Rparallelvariavel ") -> [Rparallelinput]
  [Rparallelinput] -> ?
  [Vinput3] -> ?
  TipoEntrada/1(Vu) -> [Vinput1]
  TipoEntrada/2(VuAdd) -> [Vinput2]
  TipoEntrada/3(VuRemove) -> [Vinput3]
  ? -> Mux1/1
  ConversorBoost/1(Vcoutput) -> Mux1/2
  Mux1/1 -> x/1
  ? -> Terminator/1
  ConversorBoost/2(Vu) -> Terminator1/1

== system bObserver/Slding Mode/Controlador1 ==
  note: Sinal de controle
  note: Superfície
  note: Ponto de equilíbrio
  ve : Inport
  x : Inport  Port=2
  "    " : Constant  Value=ueq
  "    2" : Constant  Value=Smep
  Constant6 : Constant  Value=boost_parameters
  Demux1 : Demux  Outputs=2
  Demux2 : Demux  Outputs=2
  Gain : Gain  Gain=0.8
  Gain1 : Gain  Gain=8
  Gain3 : Gain  Gain=2.3
  Integrator1 : Integrator
  PWM : powerlib_meascontrol/Pulse & Signal Generators/PWM Generator (DC-DC)  Fsw=7000  Ts=0
  Scope : Scope
  SlidingSurface : Subsystem
  Sum : Sum  Inputs=|++
  Sum4 : Sum  Inputs=++|
  Sum5 : Sum  Inputs=-+|
  Sum6 : Sum  Inputs=-+|
  Sum9 : Sum  Inputs=|++
  xe : MATLAB Function  TreatAsAtomicUnit=on
  sigma : Outport
  i_e : Outport  Port=2
  x_e : Outport  Port=3
  wires:
  Demux1/1 -> Sum6/2  "IL"
  PWM/1 -> sigma/1
  ve/1 -> xe/2(ve)
  Demux2/2 -> Sum5/1  "Vo1"
  "    "/1 -> Sum9/2
  Sum5/1 -> Gain3/1, Gain/1
  Sum9/1 -> PWM/1
  Demux1/2 -> Sum5/2  "Vo1"
  Demux2/1 -> Sum6/1
  xe/2(i_e) -> i_e/1
  x/1 -> Demux2/1
  Constant6/1 -> xe/1(boost_parameters)
  Gain1/1 -> Sum4/2
  xe/1(x_e) -> Demux1/1, x_e/1
  Gain/1 -> Sum/1
  Sum/1 -> Sum4/1
  SlidingSurface/1(d) -> Scope/1, Sum9/1
  "    2"/1 -> SlidingSurface/2(ep)
  Sum6/1 -> Gain1/1
  Gain3/1 -> Integrator1/1
  Integrator1/1 -> Sum/2
  Sum4/1 -> SlidingSurface/1(S)

== system bObserver/Slding Mode/D(f_s) ==
  note: iL Sensor Faults
  note: Vc Sensor Faults
  y : Inport
  Constant : Constant  Value=D1
  Constant1 : Constant  Value=VcFaultSwitch
  Constant2 : Constant  Value=iLGainFaultFactor
  Constant3 : Constant  Value=VcNoiseFaultSwitch
  Constant4 : Constant  Value=VcGainFaultFactor
  Constant7 : Constant  Value=iLFaultSwitch
  Constant8 : Constant  Value=iLNoiseFaultSwitch
  Demux : Demux  Outputs=2
  Matrix Multiply : Product  Multiplication=Matrix(*)
  Mux : Mux  Inputs=2
  Step10 : Step  Time=VcFaultTime  SampleTime=0
  Step2 : Step  Time=VcNoiseTime  SampleTime=0
  Step8 : Step  Time=iLFaultTime  SampleTime=0
  Step9 : Step  Time=iLNoiseTime  SampleTime=0
  Subsystem : Subsystem
  Subsystem2 : Subsystem
  Sum : Sum  Inputs=|+-
  y_fault : Outport
  f_s : Outport  Port=2
  wires:
  [iLoutput] -> Subsystem/1(input)
  Constant7/1 -> Subsystem/4(FaultSwtich)
  Constant8/1 -> Subsystem/5(NoiseFaultSwitch)
  Step8/1 -> Subsystem/2(FaultStep)
  Step9/1 -> Subsystem/3(NoiseStep)
  Constant1/1 -> Subsystem2/4(FaultSwtich)
  Constant3/1 -> Subsystem2/5(NoiseFaultSwitch)
  Step10/1 -> Subsystem2/2(FaultStep)
  Step2/1 -> Subsystem2/3(NoiseStep)
  Constant2/1 -> Subsystem/6(FaultFactor)
  Constant4/1 -> Subsystem2/6(FaultFactor)
  [VcOutput] -> Subsystem2/1(input)
  Demux/1 -> [iLoutput]
  Demux/2 -> [VcOutput]
  y/1 -> [y], Demux/1
  Subsystem/1(output) -> Mux/1
  Subsystem2/1(output) -> Mux/2
  Mux/1 -> Sum/2, y_fault/1
  [y] -> Sum/1
  Sum/1 -> Matrix Multiply/2
  Matrix Multiply/1 -> f_s/1
  Constant/1 -> Matrix Multiply/1  "D^- = D"

== system bObserver/Slding Mode/ErrorGenerator ==
  y_e_tilde : Inport
  y_e_tilde_hat : Inport  Port=2
  AND : Logic  IconShape=distinctive  AllPortsSameDT=off  OutDataTypeStr=boolean
  Compare To Zero : simulink/Logic and Bit Operations/Compare To Zero  relop=~=  OutDataTypeStr=boolean
  Constant1 : Constant  Value=[0;0]
  Demux : Demux  Outputs=2
  If : If  IfExpression=u1 ~= 0
  If Action Subsystem : Subsystem  TreatAsAtomicUnit=on
  If Action Subsystem1 : Subsystem  TreatAsAtomicUnit=on
  Merge : Merge  InitialOutput=[0;0]
  Sum : Sum  Inputs=|+-
  e_y : Outport
  v : Outport  Port=2
  wires:
  y_e_tilde/1 -> Sum/1
  y_e_tilde_hat/1 -> Sum/2
  Sum/1 -> Compare To Zero/1, e_y/1, [e_y]
  If/1 -> If Action Subsystem/Action
  If/2 -> If Action Subsystem1/Action
  [e_y] -> If Action Subsystem/1(e_y)
  Constant1/1 -> If Action Subsystem1/1(e_y)
  If Action Subsystem/1(v) -> Merge/1
  If Action Subsystem1/1(v) -> Merge/2
  Demux/1 -> AND/1
  Demux/2 -> AND/2
  AND/1 -> If/1
  Merge/1 -> v/1
  Compare To Zero/1 -> Demux/1

== system bObserver/Slding Mode/Fault Identification Neural Netowrk ==
  netInputs : Inport
  Constant : Constant  Commented=on  Value=MAXnet
  Constant1 : Constant  Commented=on  Value=[0;0;0]
  Constant4 : Constant  Commented=on  Value=MINnet
  Demux : Demux  Commented=on  Outputs=3
  Demux1 : Demux  Commented=on  Outputs=3
  Demux2 : Demux  Commented=on  Outputs=3
  Maximum : dspstat3/Maximum  operation=maximum  fcn=Value and Index  indexBase=One  operateOver=Each column  Dimension=1  InputProcessing=Columns as channels (frame based)  reset=None  roiEnable=off  roiType=Rectangles  roiPortion=Entire ROI  roiOutput=Individual statistics for each ROI  roiFlag=off  roundingMode=Floor  overflowMode=off  accumDataTypeStr=Inherit: Same as product output  accumLastDataTypeStr=Inherit: Same as product output
  Median Filter : dspstat3/Median Filter  Commented=on  WindowLength=1  SimulateUsing=Code generation
      settings: SourceProductBaseCode=DS
  Mux : Mux  Commented=on  Inputs=3
  Pattern Recognition Neural Network1 : Subsystem
      mask help: Pattern Recognition Neural Network
      mask Display: e = 0.06;c1 = [120 150 230]/255;c2 = ([120 150 230]+0)/383;c3 = ([120 150 230]+128)/383;patch([0 1 1 0],[0 0 1 1],c1);patch([0 1 1 1-e 1-e 0+e],[0 0 1 1-e 0+e 0+e],c2);patch([0 0 1 1-e 0+e 0+e],[0 1 1 1-e 1-e 0+e],c3);plot([0 1 1 0 0],[0 0 1 1 0]);fprintf('NNET');port_label('input',1,' Input');port_label('output',1,'Output ');
  Scope : Scope
  Scope1 : Scope
  Subsystem : Subsystem  Commented=on
  Subsystem1 : Subsystem  Commented=on
  Subsystem2 : Subsystem  Commented=on
  Terminator : Terminator
  netOutputs : Outport
  wires:
  Maximum/1 -> Terminator/1
  Maximum/2 -> Scope1/1, netOutputs/1, Scope/1
  Constant/1 -> Demux/1
  Demux2/1 -> Subsystem/1(input)
  Demux1/1 -> Subsystem/2(min)
  Demux/1 -> Subsystem/3(max)
  Demux1/2 -> Subsystem1/2(min)
  Demux/2 -> Subsystem1/3(max)
  Demux2/2 -> Subsystem1/1(input)
  Demux/3 -> Subsystem2/3(max)
  Demux1/3 -> Subsystem2/2(min)
  Demux2/3 -> Subsystem2/1(input)
  Subsystem/1(Out1) -> Mux/1
  Subsystem1/1(Out1) -> Mux/2
  Subsystem2/1(Out1) -> Mux/3
  Constant4/1 -> Demux1/1
  netInputs/1 -> Pattern Recognition Neural Network1/1(Input)
  Pattern Recognition Neural Network1/1(Output) -> Maximum/1

== system bObserver/Slding Mode/If Action Subsystem ==
  In1 : Inport
  Action Port : ActionPort  ActionPortLabel=case [ 1 6 ]:
  Out1 : Outport
  wires:
  In1/1 -> Out1/1

== system bObserver/Slding Mode/If Action Subsystem1 ==
  In1 : Inport
  Action Port : ActionPort  ActionPortLabel=default:
  Out1 : Outport
  wires:
  In1/1 -> Out1/1

== system bObserver/Slding Mode/If Action Subsystem2 ==
  y : Inport
  Action Port : ActionPort  ActionPortLabel=case [ 4 5 ]:
  x_hat : Outport
  wires:
  y/1 -> x_hat/1

== system bObserver/Slding Mode/If Action Subsystem4 ==
  y : Inport
  Action Port : ActionPort  ActionPortLabel=case [ 2 3 ]:
  x_hat : Outport
  wires:
  y/1 -> x_hat/1

== system bObserver/Slding Mode/Residual Generator2 ==
  e_y : Inport
  Matrix Square1 : dspmtrx3/Matrix Square  OutMin=[]  OutMax=[]
      settings: SourceProductBaseCode=DS
  Moving RMS : dspstat3/Moving RMS  Method=Sliding window  ForgettingFactorPort=off  SpecifyWindowLength=on  WindowLength=RMSfrequency/10  ForgettingFactor=0.9  SimulateUsing=Code generation
      settings: SourceProductBaseCode=DS
  Sqrt2 : Sqrt  SaturateOnIntegerOverflow=on
  RMS : Outport
  wires:
  Matrix Square1/1 -> Sqrt2/1
  e_y/1 -> Matrix Square1/1
  Sqrt2/1 -> Moving RMS/1
  Moving RMS/1 -> RMS/1

== system bObserver/Slding Mode/Sliding Mode Observer 5 ==
  ey : Inport
  v : Inport  Port=2
  sigma : Inport  Port=3
  C : Constant  Value=Ctilde1
  ObserverDynamics : Subsystem
  Product : Product  Multiplication=Matrix(*)
  ey_out : Outport
  y_e_tilde_hat : Outport  Port=2
  wires:
  Product/1 -> y_e_tilde_hat/1
  C/1 -> Product/1
  ObserverDynamics/1(e_tilde_hat) -> Product/2
  sigma/1 -> ObserverDynamics/3(sigma)
  ey/1 -> ey_out/1, ObserverDynamics/1(ey)
  v/1 -> ObserverDynamics/2(v)

== system bObserver/Slding Mode/Subsystem ==
  y : Inport
  C : Inport  Port=2
  y_hat : Inport  Port=3
  "    1" : Constant  Value=ObsEp
  Product : Product  Multiplication=Matrix(*)
  SlidingSurface : Subsystem
  Subtract : Sum  Inputs=+-
  error : Outport
  wires:
  Subtract/1 -> SlidingSurface/1(S)  "y-y_hat"
  Product/1 -> Subtract/1
  "    1"/1 -> SlidingSurface/2(ep)
  SlidingSurface/1(d) -> error/1
  y_hat/1 -> Subtract/2
  C/1 -> Product/1
  y/1 -> Product/2

== system bObserver/Slding Mode/Subsystem1 ==
  y : Inport
  C : Inport  Port=2
  y_hat : Inport  Port=3
  "    1" : Constant  Value=ObsEp
  Product : Product  Multiplication=Matrix(*)
  SlidingSurface : Subsystem
  Subtract : Sum  Inputs=+-
  error : Outport
  wires:
  Subtract/1 -> SlidingSurface/1(S)  "y-y_hat"
  Product/1 -> Subtract/1
  "    1"/1 -> SlidingSurface/2(ep)
  SlidingSurface/1(d) -> error/1
  y_hat/1 -> Subtract/2
  C/1 -> Product/1
  y/1 -> Product/2

== system bObserver/Slding Mode/Subsystem9 ==
  x : Inport
  Demux : Demux  Outputs=2
  Residual Generator2 : Subsystem
  Terminator : Terminator
  VcRMS : Outport
  wires:
  x/1 -> Demux/1
  Demux/2 -> Residual Generator2/1(e_y)
  Residual Generator2/1(RMS) -> VcRMS/1
  Demux/1 -> Terminator/1

== system bObserver/Slding Mode/Vc OBserver ==
  ObserverError : Inport
  C : Inport  Port=2
  sigma : Inport  Port=3
  Constant : Constant  Value=LobsVc
  Product2 : Product  Multiplication=Matrix(*)
  calc_x_hat : Subsystem
  x_hat : Outport
  y_hat : Outport  Port=2
  wires:
  sigma/1 -> calc_x_hat/1(sigma)
  calc_x_hat/1(x_hat) -> Product2/2, x_hat/1
  Product2/1 -> y_hat/1
  C/1 -> Product2/1
  ObserverError/1 -> calc_x_hat/2(rsign)
  Constant/1 -> calc_x_hat/3(Lobs)

== system bObserver/Slding Mode/iL Observer ==
  C : Inport
  ObserverError : Inport  Port=2
  sigma : Inport  Port=3
  Constant8 : Constant  Value=LobsiL
  Product2 : Product  Multiplication=Matrix(*)
  calc_x_hat : Subsystem
  x_hat : Outport
  y_hat : Outport  Port=2
  wires:
  sigma/1 -> calc_x_hat/1(sigma)
  calc_x_hat/1(x_hat) -> Product2/2, x_hat/1
  Product2/1 -> y_hat/1
  C/1 -> Product2/1
  ObserverError/1 -> calc_x_hat/2(rsign)
  Constant8/1 -> calc_x_hat/3(Lobs)
